simulink library "hal"  (Simulink 8.2)
settings: Solver=ode45  SolverMode=SingleTasking  StartTime=0.0  StopTime=10.0  RelTol=1e-3
PostLoadFcn:
  | , if any(exist('dsrtsu_mdlpostloadfcn', 'file') == [2, 3, 6]), try dsrtsu_mdlpostloadfcn('Execute', bdroot); catch fprintf('Error in PostLoadFcn (dsrtsu_mdlpostloadfcn) for model "%s":\n %s\n', bdroot, lasterr); end, end,
values from neighbouring files (symbols this model uses):
  INVALID_ABS1_TIMEOUT = single(0.03)    [hal_def.m]
  INVALID_ABS2_TIMEOUT = single(0.03)    [hal_def.m]
  INVALID_ABS3_TIMEOUT = single(0.03)    [hal_def.m]
  INVALID_ABS4_TIMEOUT = single(0.03)    [hal_def.m]
  INVALID_AC1_TIMEOUT = single(0.3)    [hal_def.m]
  INVALID_BCM1_TIMEOUT = single(0.6)    [hal_def.m]
  INVALID_BCM2_TIMEOUT = single(0.06)    [hal_def.m]
  INVALID_BOOSTER_VAC = uint32(255)    [hal_def.m]
  INVALID_CUR_VEHDECE = uint32(255)    [hal_def.m]
  INVALID_CURBRAKEDECE_REQ = uint32(255)    [hal_def.m]
  INVALID_CURSTEERANG_REQ = uint32(65535)    [hal_def.m]
  INVALID_CURSTEERTQ_REQ = uint32(255)    [hal_def.m]
  INVALID_ECM1_TIMEOUT = single(0.03)    [hal_def.m]
  INVALID_ECM2_TIMEOUT = single(0.03)    [hal_def.m]
  INVALID_ECM3_TIMEOUT = single(0.03)    [hal_def.m]
  INVALID_ECM9_TIMEOUT = single(0.03)    [hal_def.m]
  INVALID_ENG_TORQUE_FRICTIONAL = uint32(255)    [hal_def.m]
  INVALID_ENG_TORQUE_INDICATED = uint32(255)    [hal_def.m]
  INVALID_ENG_TORQUE_INDICATEDCOR = uint32(255)    [hal_def.m]
  INVALID_ENG_TQ_MAX = uint32(65535)    [hal_def.m]
  INVALID_ENG_TQ_MIN = uint32(65535)    [hal_def.m]
  INVALID_EPAS2_TIMEOUT = single(0.03)    [hal_def.m]
  INVALID_EPAS3_TIMEOUT = single(0.03)    [hal_def.m]
  INVALID_EPB1_TIMEOUT = single(0.12)    [hal_def.m]
  INVALID_EPS_BATTVOLT = uint32(251)    [hal_def.m]
  INVALID_ESC_BATTVOLT = uint32(251)    [hal_def.m]
  INVALID_GRADE = uint32(255)    [hal_def.m]
  INVALID_HCU3_TIMEOUT = single(0.03)    [hal_def.m]
  INVALID_HCU4_TIMEOUT = single(0.03)    [hal_def.m]
  INVALID_HMI1_TIMEOUT = single(0.03)    [hal_def.m]
  INVALID_HMI2_TIMEOUT = single(0.03)    [hal_def.m]
  INVALID_LAT_ACC = uint32(255)    [hal_def.m]
  INVALID_LONG_ACC = uint32(255)    [hal_def.m]
  INVALID_MC_PRESSURE = uint32(2047)    [hal_def.m]
  INVALID_METER1_TIMEOUT = single(0.3)    [hal_def.m]
  INVALID_METER3_TIMEOUT = single(0.3)    [hal_def.m]
  INVALID_METER_VEHSPD = uint32(2048)    [hal_def.m]
  INVALID_ODO_METER = uint32(1000000)    [hal_def.m]
  INVALID_OUTSIDE_TEMP = uint32(96)    [hal_def.m]
  INVALID_PARKBRAKEBIND_STAT = uint32(3)    [hal_def.m]
  INVALID_SAS1_TIMEOUT = single(0.03)    [hal_def.m]
  INVALID_SAS_ANGLE = uint32(65535)    [hal_def.m]
  INVALID_SHIFTER_POSN = uint32(6)    [hal_def.m]
  INVALID_TCM1_TIMEOUT = single(0.03)    [hal_def.m]
  INVALID_TCM2_TIMEOUT = single(0.03)    [hal_def.m]
  INVALID_VCU1_TIMEOUT = single(0.03)    [hal_def.m]
  INVALID_VCU2_TIMEOUT = single(0.03)    [hal_def.m]
  INVALID_VEH_CRASH = uint32(15)    [hal_def.m]
  INVALID_VEH_SPD = uint32(2048)    [hal_def.m]
  INVALID_WHEEL_SPD = uint32(16377)    [hal_def.m]
  INVALID_YAW_RATE = uint32(2001)    [hal_def.m]
undefined symbols (not defined in the file or in its folder): C_TASK_5MS_S, FALSE, INVALID_CURPTTORQ_REQ, KHAL_MssgIdObj1_num, KHAL_MssgIdObj2_num, KHAL_MssgIdObjStatus_num, TRUE
libraries: simulink x92
(part 7 of 8)

== system hal/dHAL_IN/HAL_IN_VCU/BO__883_HCU3__8_VCU ==
  CAN1_Rx : Inport
  Bus Selector : BusSelector  OutputSignals=HCU3.EngTqIndPermMax,HCU3.EngTqIndPermMax_P,HCU3.HCU3RollCnt
  EngTqIndPermMax : Outport
  EngTqIndPermMax_P : Outport  Port=2
  HCU3RollCnt : Outport  Port=3
  wires:
  Bus Selector/1 -> EngTqIndPermMax/1  "<EngTqIndPermMax>"
  Bus Selector/3 -> HCU3RollCnt/1  "<HCU3RollCnt>"
  Bus Selector/2 -> EngTqIndPermMax_P/1  "<EngTqIndPermMax_P>"
  [CAN1_Rx] -> Bus Selector/1
  CAN1_Rx/1 -> [CAN1_Rx]

== system hal/dHAL_IN/HAL_IN_VCU/BO__899_HCU4__8_VCU ==
  CAN1_Rx : Inport
  Bus Selector : BusSelector  OutputSignals=HCU4.MILReq
  MILReq : Outport
  wires:
  Bus Selector/1 -> MILReq/1  "<MILReq>"
  CAN1_Rx/1 -> [CAN1_Rx]
  [CAN1_Rx] -> Bus Selector/1

== system hal/dHAL_IN/dHAL_IN_ABS/BO_864_ABS2_8_ABS ==
  CAN1_Rx : Inport
  Bitwise Operator : simulink/Logic and Bit Operations/Bitwise Operator  logicop=AND  UseBitMask=on  BitMask=bin2dec('11110000')  BitMaskRealWorld=Stored Integer
  Bus Selector : BusSelector  OutputSignals=ABS2.ABS_Active,ABS2.ABS_Failed,ABS2.BrkSw_Sta,ABS2.BrkSw_V,ABS2.EBD_Failed,ABS2.ESC_Active,ABS2.ESC_Failed,ABS2.HSA_Active,ABS2.HSA_Failed,ABS2.TCS_Active,ABS2.TCS_Enabled,ABS2.TCS_Failed,ABS2.VehSpeed,ABS2.VehSpeed_Checksum,ABS2.VehSpeed_LifeCount
  Bus Selector1 : BusSelector  OutputSignals=ABS2.RAW_Byte_2,ABS2.RAW_Byte_1
  ChecksumCalculation : Subsystem  TreatAsAtomicUnit=on
  IcM : Subsystem  TreatAsAtomicUnit=on
  ABS_Active : Outport
  ABS_Failed : Outport  Port=2
  BrkSw_Sta : Outport  Port=3
  BrkSw_V : Outport  Port=4
  EBD_Failed : Outport  Port=5
  ESC_Active : Outport  Port=6
  ESC_Failed : Outport  Port=7
  HSA_Active : Outport  Port=8
  HSA_Failed : Outport  Port=9
  TCS_Active : Outport  Port=10
  TCS_Enabled : Outport  Port=11
  TCS_Failed : Outport  Port=12
  VehSpeed : Outport  Port=13
  VehSpeed_raw : Outport  Port=14
  VehSpeed_LifeCount : Outport  Port=15
  VehSpeed_Checksum : Outport  Port=16
  Message_Checksum : Outport  Port=17
  wires:
  IcM/1(HighLowByte) -> VehSpeed_raw/1
  Bitwise Operator/1 -> IcM/1(LowByte)
  Bus Selector1/2 -> IcM/2(HighByte)  "<RAW_Byte_1>"
  Bus Selector1/1 -> Bitwise Operator/1  "<RAW_Byte_2>"
  [CAN1_Rx] -> Bus Selector1/1
  ChecksumCalculation/1(Message_Checksum) -> Message_Checksum/1
  [CAN1_Rx] -> ChecksumCalculation/1(CAN1_Rx)
  Bus Selector/15 -> VehSpeed_LifeCount/1  "<VehSpeed_LifeCount>"
  Bus Selector/14 -> VehSpeed_Checksum/1  "<VehSpeed_Checksum>"
  Bus Selector/13 -> VehSpeed/1  "<VehSpeed>"
  Bus Selector/12 -> TCS_Failed/1  "<TCS_Failed>"
  Bus Selector/11 -> TCS_Enabled/1  "<TCS_Enabled>"
  Bus Selector/10 -> TCS_Active/1  "<TCS_Active>"
  Bus Selector/9 -> HSA_Failed/1  "<HSA_Failed>"
  Bus Selector/8 -> HSA_Active/1  "<HSA_Active>"
  Bus Selector/7 -> ESC_Failed/1  "<ESC_Failed>"
  Bus Selector/6 -> ESC_Active/1  "<ESC_Active>"
  Bus Selector/5 -> EBD_Failed/1  "<EBD_Failed>"
  Bus Selector/4 -> BrkSw_V/1  "<BrkSw_V>"
  Bus Selector/3 -> BrkSw_Sta/1  "<BrkSw_Sta>"
  Bus Selector/2 -> ABS_Failed/1  "<ABS_Failed>"
  Bus Selector/1 -> ABS_Active/1  "<ABS_Active>"
  CAN1_Rx/1 -> [CAN1_Rx]
  [CAN1_Rx] -> Bus Selector/1

== system hal/dHAL_IN/dHAL_IN_ABS/BO__848_ABS1__8_ABS ==
  CAN1_Rx : Inport
  Bus Selector : BusSelector  OutputSignals=ABS1.BoosterVac,ABS1.BoosterVac_Failed,ABS1.BoosterVac_Sta,ABS1.BoosterVac_V,ABS1.GRADE,ABS1.GRADE_V,ABS1.TCSRollCnt
  Bus Selector1 : BusSelector  OutputSignals=ABS1.RAW_Byte_8,ABS1.RAW_Byte_7
  BoosterVac : Outport
  BoosterVac_raw : Outport  Port=2
  BoosterVac_V : Outport  Port=3
  BoosterVac_Sta : Outport  Port=4
  BoosterVac_Failed : Outport  Port=5
  GRADE : Outport  Port=6
  GRADE_raw : Outport  Port=7
  GRADE_V : Outport  Port=8
  TCSRollCnt : Outport  Port=9
  wires:
  Bus Selector1/2 -> GRADE_raw/1  "<RAW_Byte_7>"
  Bus Selector1/1 -> BoosterVac_raw/1  "<RAW_Byte_8>"
  [CAN1_Rx] -> Bus Selector1/1
  Bus Selector/7 -> TCSRollCnt/1  "<TCSRollCnt>"
  Bus Selector/6 -> GRADE_V/1  "<GRADE_V>"
  Bus Selector/5 -> GRADE/1  "<GRADE>"
  Bus Selector/4 -> BoosterVac_V/1  "<BoosterVac_V>"
  Bus Selector/3 -> BoosterVac_Sta/1  "<BoosterVac_Sta>"
  Bus Selector/2 -> BoosterVac_Failed/1  "<BoosterVac_Failed>"
  Bus Selector/1 -> BoosterVac/1  "<BoosterVac>"
  CAN1_Rx/1 -> [CAN1_Rx]
  [CAN1_Rx] -> Bus Selector/1

== system hal/dHAL_IN/dHAL_IN_ABS/BO__880_ABS3__8_ABS ==
  CAN1_Rx : Inport
  Bitwise Operator{,1..3} (4 alike) : simulink/Logic and Bit Operations/Bitwise Operator  logicop=AND  UseBitMask=on  BitMask=bin2dec('11111110')  BitMaskRealWorld=Stored Integer
  Bus Selector : BusSelector  OutputSignals=ABS3.LF_RawWhlSpeed,ABS3.LF_RawWhlSpeed_V,ABS3.LR_RawWhlSpeed,ABS3.LR_RawWhlSpeed_V,ABS3.RF_RawWhlSpeed,ABS3.RF_RawWhlSpeed_V,ABS3.RR_RawWhlSpeed,ABS3.RR_RawWhlSpeed_V
  Bus Selector1 : BusSelector  OutputSignals=ABS3.RAW_Byte_2,ABS3.RAW_Byte_1,ABS3.RAW_Byte_4,ABS3.RAW_Byte_3,ABS3.RAW_Byte_6,ABS3.RAW_Byte_5,ABS3.RAW_Byte_8,ABS3.RAW_Byte_7
  IcM : Subsystem  TreatAsAtomicUnit=on
  IcM1 : Subsystem  TreatAsAtomicUnit=on
  IcM2 : Subsystem  TreatAsAtomicUnit=on
  IcM3 : Subsystem  TreatAsAtomicUnit=on
  LF_RawWhlSpeed : Outport
  LF_RawWhlSpeed_raw : Outport  Port=2
  LF_RawWhlSpeed_V : Outport  Port=3
  LR_RawWhlSpeed : Outport  Port=4
  LR_RawWhlSpeed_raw : Outport  Port=5
  LR_RawWhlSpeed_V : Outport  Port=6
  RF_RawWhlSpeed : Outport  Port=7
  RF_RawWhlSpeed_raw : Outport  Port=8
  RF_RawWhlSpeed_V : Outport  Port=9
  RR_RawWhlSpeed : Outport  Port=10
  RR_RawWhlSpeed_raw : Outport  Port=11
  RR_RawWhlSpeed_V : Outport  Port=12
  wires:
  IcM3/1(HighLowByte) -> LF_RawWhlSpeed_raw/1
  IcM2/1(HighLowByte) -> RF_RawWhlSpeed_raw/1
  Bus Selector1/8 -> IcM3/2(HighByte)  "<RAW_Byte_7>"
  Bus Selector1/7 -> Bitwise Operator3/1  "<RAW_Byte_8>"
  Bus Selector1/6 -> IcM2/2(HighByte)  "<RAW_Byte_5>"
  Bus Selector1/5 -> Bitwise Operator2/1  "<RAW_Byte_6>"
  Bitwise Operator3/1 -> IcM3/1(LowByte)
  Bitwise Operator2/1 -> IcM2/1(LowByte)
  Bus Selector1/4 -> IcM1/2(HighByte)  "<RAW_Byte_3>"
  Bus Selector1/3 -> Bitwise Operator1/1  "<RAW_Byte_4>"
  IcM1/1(HighLowByte) -> LR_RawWhlSpeed_raw/1
  Bitwise Operator1/1 -> IcM1/1(LowByte)
  Bus Selector1/2 -> IcM/2(HighByte)  "<RAW_Byte_1>"
  Bus Selector1/1 -> Bitwise Operator/1  "<RAW_Byte_2>"
  IcM/1(HighLowByte) -> RR_RawWhlSpeed_raw/1
  Bitwise Operator/1 -> IcM/1(LowByte)
  [CAN1_Rx] -> Bus Selector1/1
  Bus Selector/8 -> RR_RawWhlSpeed_V/1  "<RR_RawWhlSpeed_V>"
  Bus Selector/7 -> RR_RawWhlSpeed/1  "<RR_RawWhlSpeed>"
  Bus Selector/6 -> RF_RawWhlSpeed_V/1  "<RF_RawWhlSpeed_V>"
  Bus Selector/5 -> RF_RawWhlSpeed/1  "<RF_RawWhlSpeed>"
  Bus Selector/4 -> LR_RawWhlSpeed_V/1  "<LR_RawWhlSpeed_V>"
  Bus Selector/3 -> LR_RawWhlSpeed/1  "<LR_RawWhlSpeed>"
  Bus Selector/2 -> LF_RawWhlSpeed_V/1  "<LF_RawWhlSpeed_V>"
  Bus Selector/1 -> LF_RawWhlSpeed/1  "<LF_RawWhlSpeed>"
  [CAN1_Rx] -> Bus Selector/1
  CAN1_Rx/1 -> [CAN1_Rx]

== system hal/dHAL_IN/dHAL_IN_ABS/BO__896_ABS4__8_ABS ==
  CAN1_Rx : Inport
  Bitwise Operator : simulink/Logic and Bit Operations/Bitwise Operator  logicop=AND  UseBitMask=on  BitMask=bin2dec('00000111')  BitMaskRealWorld=Stored Integer
  Bus Selector : BusSelector  OutputSignals=ABS4.LatAccel,ABS4.LatAccel_V,ABS4.LongAccel,ABS4.LongAccel_V,ABS4.MCPressure,ABS4.MCPressure_V,ABS4.YawRate,ABS4.YawRate_V
  Bus Selector1 : BusSelector  OutputSignals=ABS4.RAW_Byte_3,ABS4.RAW_Byte_8,ABS4.RAW_Byte_5,ABS4.RAW_Byte_4
  Bus Selector2 : BusSelector  OutputSignals=ABS4.RAW_Byte_2,ABS4.RAW_Byte_1
  IcM : Subsystem  TreatAsAtomicUnit=on
  IcM1 : Subsystem  TreatAsAtomicUnit=on
  LatAccel : Outport
  LatAccel_raw : Outport  Port=2
  LatAccel_V : Outport  Port=3
  LongAccel : Outport  Port=4
  LongAcce_raw : Outport  Port=5
  LongAccel_V : Outport  Port=6
  MCPressure : Outport  Port=7
  MCPressure_raw : Outport  Port=8
  MCPressure_V : Outport  Port=9
  YawRate : Outport  Port=10
  YawRate_raw : Outport  Port=11
  YawRate_V : Outport  Port=12
  wires:
  Bitwise Operator/1 -> IcM1/2(HighByte)
  Bus Selector2/2 -> Bitwise Operator/1  "<RAW_Byte_1>"
  Bus Selector2/1 -> IcM1/1(LowByte)  "<RAW_Byte_2>"
  IcM/1(HighLowByte) -> YawRate_raw/1
  IcM1/1(HighLowByte) -> MCPressure_raw/1
  [CAN1_Rx] -> Bus Selector2/1
  Bus Selector1/4 -> IcM/2(HighByte)  "<RAW_Byte_4>"
  Bus Selector1/3 -> IcM/1(LowByte)  "<RAW_Byte_5>"
  Bus Selector1/2 -> LongAcce_raw/1  "<RAW_Byte_8>"
  Bus Selector1/1 -> LatAccel_raw/1  "<RAW_Byte_3>"
  [CAN1_Rx] -> Bus Selector1/1
  Bus Selector/8 -> YawRate_V/1  "<YawRate_V>"
  Bus Selector/7 -> YawRate/1  "<YawRate>"
  Bus Selector/6 -> MCPressure_V/1  "<MCPressure_V>"
  Bus Selector/5 -> MCPressure/1  "<MCPressure>"
  Bus Selector/4 -> LongAccel_V/1  "<LongAccel_V>"
  Bus Selector/3 -> LongAccel/1  "<LongAccel>"
  Bus Selector/2 -> LatAccel_V/1  "<LatAccel_V>"
  Bus Selector/1 -> LatAccel/1  "<LatAccel>"
  [CAN1_Rx] -> Bus Selector/1
  CAN1_Rx/1 -> [CAN1_Rx]

== system hal/dHAL_IN/dHAL_IN_AC/BO__1120_AC1__8_AC ==
  CAN1_Rx : Inport
  Bus Selector : BusSelector  OutputSignals=AC1.Sta_Out_Temp
  Bus Selector1 : BusSelector  OutputSignals=AC1.RAW_Byte_8
  Sta_Out_Temp : Outport
  Sta_Out_Temp_raw : Outport  Port=2
  wires:
  Bus Selector1/1 -> Sta_Out_Temp_raw/1  "<RAW_Byte_8>"
  Bus Selector/1 -> Sta_Out_Temp/1  "<Sta_Out_Temp>"
  [CAN1_Rx] -> Bus Selector1/1
  CAN1_Rx/1 -> [CAN1_Rx]
  [CAN1_Rx] -> Bus Selector/1

== system hal/dHAL_IN/dHAL_IN_BCM/BO__1008_BCM2__8_BCM ==
  CAN1_Rx : Inport
  Bus Selector : BusSelector  OutputSignals=BCM2.BCM_SRS_Crash_Info
  BCM_SRS_Crash_Info : Outport
  wires:
  Bus Selector/1 -> BCM_SRS_Crash_Info/1  "<BCM_SRS_Crash_Info>"
  CAN1_Rx/1 -> [CAN1_Rx]
  [CAN1_Rx] -> Bus Selector/1

== system hal/dHAL_IN/dHAL_IN_BCM/BO__1056_BCM1__8_BCM ==
  CAN1_Rx : Inport
  Bus Selector : BusSelector  OutputSignals=BCM1.BCM_AllDrSw_Sta,BCM1.BCM_DDrSw_Sta,BCM1.BCM_Hazard_Sta,BCM1.BCM_Key_Sta,BCM1.BCM_LRDrSw_Sta,BCM1.BCM_LTurnLp_Sta,BCM1.BCM_PDrSw_Sta,BCM1.BCM_RRDrSw_Sta,BCM1.BCM_RTurnLp_Sta,BCM1.BCM_TGateSw_Sta
  BCM_AllDrSw_Sta : Outport
  BCM_DDrSw_Sta : Outport  Port=2
  BCM_Hazard_Sta : Outport  Port=3
  BCM_Key_Sta : Outport  Port=4
  BCM_LRDrSw_Sta : Outport  Port=5
  BCM_LTurnLp_Sta : Outport  Port=6
  BCM_PDrSw_Sta : Outport  Port=7
  BCM_RRDrSw_Sta : Outport  Port=8
  BCM_RTurnLp_Sta : Outport  Port=9
  BCM_TGateSw_Sta : Outport  Port=10
  wires:
  Bus Selector/10 -> BCM_TGateSw_Sta/1  "<BCM_TGateSw_Sta>"
  Bus Selector/9 -> BCM_RTurnLp_Sta/1  "<BCM_RTurnLp_Sta>"
  Bus Selector/8 -> BCM_RRDrSw_Sta/1  "<BCM_RRDrSw_Sta>"
  Bus Selector/7 -> BCM_PDrSw_Sta/1  "<BCM_PDrSw_Sta>"
  Bus Selector/6 -> BCM_LTurnLp_Sta/1  "<BCM_LTurnLp_Sta>"
  Bus Selector/5 -> BCM_LRDrSw_Sta/1  "<BCM_LRDrSw_Sta>"
  Bus Selector/4 -> BCM_Key_Sta/1  "<BCM_Key_Sta>"
  Bus Selector/3 -> BCM_Hazard_Sta/1  "<BCM_Hazard_Sta>"
  Bus Selector/2 -> BCM_DDrSw_Sta/1  "<BCM_DDrSw_Sta>"
  Bus Selector/1 -> BCM_AllDrSw_Sta/1  "<BCM_AllDrSw_Sta>"
  [CAN1_Rx] -> Bus Selector/1
  CAN1_Rx/1 -> [CAN1_Rx]

== system hal/dHAL_IN/dHAL_IN_ECM/BO_790_ECM1_8_ECM ==
  CAN1_Rx : Inport
  Bus Selector : BusSelector  OutputSignals=ECM1.CAN_N,ECM1.CAN_TQFR,ECM1.CAN_TQI,ECM1.CAN_TQI_ACOR,ECM1.CAN_TQ_STND,ECM1.LV_CAN_N_ERR,ECM1.LV_CAN_SUB_TQI
  Bus Selector1 : BusSelector  OutputSignals=ECM1.RAW_Byte_6,ECM1.RAW_Byte_5,ECM1.RAW_Byte_2
  CAN_N : Outport
  CAN_TQFR : Outport  Port=2
  CAN_TQFR_raw : Outport  Port=3
  CAN_TQI : Outport  Port=4
  CAN_TQI_raw : Outport  Port=5
  CAN_TQI_ACOR : Outport  Port=6
  CAN_TQI_ACOR_raw : Outport  Port=7
  CAN_TQ_STND : Outport  Port=8
  LV_CAN_N_ERR : Outport  Port=9
  LV_CAN_SUB_TQI : Outport  Port=10
  wires:
  [CAN1_Rx] -> Bus Selector1/1
  [CAN1_Rx] -> Bus Selector/1
  CAN1_Rx/1 -> [CAN1_Rx]
  Bus Selector1/3 -> CAN_TQI_ACOR_raw/1  "<RAW_Byte_2>"
  Bus Selector1/2 -> CAN_TQI_raw/1  "<RAW_Byte_5>"
  Bus Selector1/1 -> CAN_TQFR_raw/1  "<RAW_Byte_6>"
  Bus Selector/7 -> LV_CAN_SUB_TQI/1  "<LV_CAN_SUB_TQI>"
  Bus Selector/6 -> LV_CAN_N_ERR/1  "<LV_CAN_N_ERR>"
  Bus Selector/5 -> CAN_TQ_STND/1  "<CAN_TQ_STND>"
  Bus Selector/4 -> CAN_TQI_ACOR/1  "<CAN_TQI_ACOR>"
  Bus Selector/3 -> CAN_TQI/1  "<CAN_TQI>"
  Bus Selector/2 -> CAN_TQFR/1  "<CAN_TQFR>"
  Bus Selector/1 -> CAN_N/1  "<CAN_N>"

== system hal/dHAL_IN/dHAL_IN_ECM/BO_809_ECM2_8_ECM ==
  CAN1_Rx : Inport
  Bus Selector : BusSelector  OutputSignals=ECM2.Eng_Hood_SW,ECM2.LV_CAN_ENG_RUN_ST
  Eng_Hood_SW : Outport
  LV_CAN_ENG_RUN_ST : Outport  Port=2
  wires:
  Bus Selector/1 -> Eng_Hood_SW/1  "<Eng_Hood_SW>"
  Bus Selector/2 -> LV_CAN_ENG_RUN_ST/1  "<LV_CAN_ENG_RUN_ST>"
  CAN1_Rx/1 -> Bus Selector/1

== system hal/dHAL_IN/dHAL_IN_ECM/BO_821_ECM3_8_ECM ==
  CAN1_Rx : Inport
  Bus Selector : BusSelector  OutputSignals=ECM3.CAN_PV_AV,ECM3.CAN_PV_EFC,ECM3.LV_CAN_ERRPAS,ECM3.LV_CAN_ERRPVS,ECM3.LV_CAN_MAIN_CRU,ECM3.LV_CAN_MAIN_CRU_ER,ECM3.LV_CAN_SET_CRU,ECM3.LV_CAN_SET_CRU_ERR
  CAN_PV_AV : Outport
  CAN_PV_EFC : Outport  Port=2
  LV_CAN_ERRPAS : Outport  Port=3
  LV_CAN_ERRPVS : Outport  Port=4
  LV_CAN_MAIN_CRU : Outport  Port=5
  LV_CAN_MAIN_CRU_ER : Outport  Port=6
  LV_CAN_SET_CRU : Outport  Port=7
  LV_CAN_SET_CRU_ERR : Outport  Port=8
  wires:
  Bus Selector/8 -> LV_CAN_SET_CRU_ERR/1  "<LV_CAN_SET_CRU_ERR>"
  Bus Selector/7 -> LV_CAN_SET_CRU/1  "<LV_CAN_SET_CRU>"
  Bus Selector/6 -> LV_CAN_MAIN_CRU_ER/1  "<LV_CAN_MAIN_CRU_ER>"
  Bus Selector/5 -> LV_CAN_MAIN_CRU/1  "<LV_CAN_MAIN_CRU>"
  Bus Selector/4 -> LV_CAN_ERRPVS/1  "<LV_CAN_ERRPVS>"
  Bus Selector/3 -> LV_CAN_ERRPAS/1  "<LV_CAN_ERRPAS>"
  Bus Selector/2 -> CAN_PV_EFC/1  "<CAN_PV_EFC>"
  Bus Selector/1 -> CAN_PV_AV/1  "<CAN_PV_AV>"
  CAN1_Rx/1 -> Bus Selector/1

== system hal/dHAL_IN/dHAL_IN_ECM/BO_875_ECM9_8_ECM ==
  CAN1_Rx1 : Inport
  Bus Selector : BusSelector  OutputSignals=ECM9.ECM9RollCnt,ECM9.EMSHybridOpState,ECM9.EMSOpState,ECM9.EngTqMax,ECM9.EngTqMin
  Bus Selector1 : BusSelector  OutputSignals=ECM9.RAW_Byte_5,ECM9.RAW_Byte_4,ECM9.RAW_Byte_7,ECM9.RAW_Byte_6
  IcM : Subsystem  TreatAsAtomicUnit=on
  IcM1 : Subsystem  TreatAsAtomicUnit=on
  ECM9RollCnt : Outport
  EMSHybridOpState : Outport  Port=2
  EMSOpState : Outport  Port=3
  EngTqMax : Outport  Port=4
  EngTqMax_raw : Outport  Port=5
  EngTqMin : Outport  Port=6
  EngTqMin_raw : Outport  Port=7
  wires:
  [CAN1_Rx] -> Bus Selector1/1
  [CAN1_Rx] -> Bus Selector/1
  CAN1_Rx1/1 -> [CAN1_Rx]
  IcM1/1(HighLowByte) -> EngTqMin_raw/1
  IcM/1(HighLowByte) -> EngTqMax_raw/1
  Bus Selector1/4 -> IcM1/2(HighByte)  "<RAW_Byte_6>"
  Bus Selector1/3 -> IcM1/1(LowByte)  "<RAW_Byte_7>"
  Bus Selector1/2 -> IcM/2(HighByte)  "<RAW_Byte_4>"
  Bus Selector1/1 -> IcM/1(LowByte)  "<RAW_Byte_5>"
  Bus Selector/5 -> EngTqMin/1  "<EngTqMin>"
  Bus Selector/4 -> EngTqMax/1  "<EngTqMax>"
  Bus Selector/3 -> EMSOpState/1  "<EMSOpState>"
  Bus Selector/2 -> EMSHybridOpState/1  "<EMSHybridOpState>"
  Bus Selector/1 -> ECM9RollCnt/1  "<ECM9RollCnt>"

== system hal/dHAL_IN/dHAL_IN_EPAS/BO__1365_EPAS3__8_EPAS ==
  CAN1_Rx : Inport
  Bus Selector : BusSelector  OutputSignals=EPAS3.CurStrAngReq,EPAS3.CurStrTqReq_A,EPAS3.CurStrTqReq,EPAS3.CurStrTqReq_A,EPAS3.DriverStrIntd,EPAS3.DriverStrIntdLvl,EPAS3.EPSBattVolt,EPAS3.EPAS3_Checksum,EPAS3.EPAS3_LifeCount
  Bus Selector1 : BusSelector  OutputSignals=EPAS3.RAW_Byte_2,EPAS3.RAW_Byte_1,EPAS3.RAW_Byte_5,EPAS3.RAW_Byte_6
  ChecksumCalculation : Subsystem  TreatAsAtomicUnit=on
  IcM : Subsystem  TreatAsAtomicUnit=on
  CurStrAngReq : Outport
  CurStrAngReq_raw : Outport  Port=2
  CurStrAngReq_A : Outport  Port=3
  CurStrTqReq : Outport  Port=4
  CurStrTqReq_raw : Outport  Port=5
  CurStrTqReq_A : Outport  Port=6
  DriverStrIntd : Outport  Port=7
  DriverStrIntdLvl : Outport  Port=8
  EPAS3_LifeCount : Outport  Port=9
  EPSBattVolt : Outport  Port=10
  EPSBattVolt_raw : Outport  Port=11
  EPAS3_Checksum : Outport  Port=12
  Message_Checksum : Outport  Port=13
  wires:
  Bus Selector1/4 -> EPSBattVolt_raw/1  "<RAW_Byte_6>"
  Bus Selector1/3 -> CurStrTqReq_raw/1  "<RAW_Byte_5>"
  IcM/1(HighLowByte) -> CurStrAngReq_raw/1
  Bus Selector1/2 -> IcM/2(HighByte)  "<RAW_Byte_1>"
  Bus Selector1/1 -> IcM/1(LowByte)  "<RAW_Byte_2>"
  Bus Selector/4 -> CurStrTqReq_A/1  "<CurStrTqReq_A>"
  Bus Selector/2 -> CurStrAngReq_A/1  "<CurStrTqReq_A>"
  ChecksumCalculation/1(Message_Checksum) -> Message_Checksum/1
  Bus Selector/7 -> EPSBattVolt/1  "<EPSBattVolt>"
  Bus Selector/9 -> ChecksumCalculation/1(EPAS3_LifeCount), EPAS3_LifeCount/1  "<EPAS3_LifeCount>"
  Bus Selector/8 -> EPAS3_Checksum/1  "<EPAS3_Checksum>"
  Bus Selector/6 -> DriverStrIntdLvl/1  "<DriverStrIntdLvl>"
  Bus Selector/5 -> DriverStrIntd/1  "<DriverStrIntd>"
  Bus Selector/3 -> CurStrTqReq/1  "<CurStrTqReq>"
  Bus Selector/1 -> CurStrAngReq/1  "<CurStrAngReq>"
  [CAN1_Rx] -> Bus Selector/1
  CAN1_Rx/1 -> [CAN1_Rx]
  [CAN1_Rx] -> ChecksumCalculation/2(CAN1_Rx)
  [CAN1_Rx] -> Bus Selector1/1

== system hal/dHAL_IN/dHAL_IN_EPAS/BO__922_SAS1__8_EPAS ==
  CAN1_Rx : Inport
  Bus Selector : BusSelector  OutputSignals=SAS1.SAS_Angle,SAS1.SAS_CAL,SAS1.SAS_CheckSum,SAS1.SAS_OK,SAS1.SAS_MsgCount
  Bus Selector1 : BusSelector  OutputSignals=SAS1.RAW_Byte_2,SAS1.RAW_Byte_1
  ChecksumCalculation : Subsystem  TreatAsAtomicUnit=on
  IcM : Subsystem  TreatAsAtomicUnit=on
  SAS_Angle : Outport
  SAS_Angle_raw : Outport  Port=2
  SAS_CAL : Outport  Port=3
  SAS_OK : Outport  Port=4
  SAS_MsgCount : Outport  Port=5
  SAS_CheckSum : Outport  Port=6
  Message_Checksum : Outport  Port=7
  wires:
  IcM/1(HighLowByte) -> SAS_Angle_raw/1
  Bus Selector1/2 -> IcM/2(HighByte)  "<RAW_Byte_1>"
  Bus Selector1/1 -> IcM/1(LowByte)  "<RAW_Byte_2>"
  [CAN1_Rx] -> Bus Selector1/1
  [CAN1_Rx] -> ChecksumCalculation/2(CAN1_Rx)
  ChecksumCalculation/1(Message_Checksum) -> Message_Checksum/1
  Bus Selector/4 -> SAS_OK/1  "<SAS_OK>"
  Bus Selector/5 -> ChecksumCalculation/1(SAS_MsgCount), SAS_MsgCount/1  "<SAS_MsgCount>"
  Bus Selector/3 -> SAS_CheckSum/1  "<SAS_CheckSum>"
  Bus Selector/2 -> SAS_CAL/1  "<SAS_CAL>"
  Bus Selector/1 -> SAS_Angle/1  "<SAS_Angle>"
  [CAN1_Rx] -> Bus Selector/1
  CAN1_Rx/1 -> [CAN1_Rx]

== system hal/dHAL_IN/dHAL_IN_EPAS/BO__926_EPAS2__8_EPAS ==
  CAN1_Rx : Inport
  Bus Selector : BusSelector  OutputSignals=EPAS2.Elect_PWR_Consumpt,EPAS2.EpasFailed,EPAS2.RSP_OK,EPAS2.R_SAS_Angle,EPAS2.Steering_Torque,EPAS2.Steering_Torque_V,EPAS2.SAS_CheckSum2,EPAS2.SAS_MsgCount2
  Bus Selector1 : BusSelector  OutputSignals=EPAS2.RAW_Byte_5,EPAS2.RAW_Byte_4
  ChecksumCalculation : Subsystem  TreatAsAtomicUnit=on
  IcM : Subsystem  TreatAsAtomicUnit=on
  Elect_PWR_Consumpt : Outport
  EpasFailed : Outport  Port=2
  R_SAS_Angle : Outport  Port=3
  R_SAS_Angle_raw : Outport  Port=4
  RSP_OK : Outport  Port=5
  SAS_MsgCount2 : Outport  Port=6
  Steering_Torque : Outport  Port=7
  Steering_Torque_V : Outport  Port=8
  SAS_CheckSum2 : Outport  Port=9
  Message_Checksum : Outport  Port=10
  wires:
  IcM/1(HighLowByte) -> R_SAS_Angle_raw/1
  Bus Selector1/2 -> IcM/2(HighByte)  "<RAW_Byte_4>"
  Bus Selector1/1 -> IcM/1(LowByte)  "<RAW_Byte_5>"
  [CAN1_Rx] -> Bus Selector1/1
  [CAN1_Rx] -> ChecksumCalculation/2(CAN1_Rx)
  ChecksumCalculation/1(Message_Checksum) -> Message_Checksum/1
  Bus Selector/6 -> Steering_Torque_V/1  "<Steering_Torque_V>"
  Bus Selector/5 -> Steering_Torque/1  "<Steering_Torque>"
  Bus Selector/8 -> SAS_MsgCount2/1, ChecksumCalculation/1(SAS_MsgCount)  "<SAS_MsgCount2>"
  Bus Selector/7 -> SAS_CheckSum2/1  "<SAS_CheckSum2>"
  Bus Selector/4 -> R_SAS_Angle/1  "<R_SAS_Angle>"
  Bus Selector/3 -> RSP_OK/1  "<RSP_OK>"
  Bus Selector/2 -> EpasFailed/1  "<EpasFailed>"
  Bus Selector/1 -> Elect_PWR_Consumpt/1  "<Elect_PWR_Consumpt>"
  CAN1_Rx/1 -> [CAN1_Rx]
  [CAN1_Rx] -> Bus Selector/1

== system hal/dHAL_IN/dHAL_IN_METER/BO__1104_Meter1__8_Meter ==
  CAN1_Rx : Inport
  Bus Selector : BusSelector  OutputSignals=Meter1.LowBrakeFluid_Sta,Meter1.ODOMETER,Meter1.ParkBrake,Meter1.SeatBelt
  LowBrakeFluid_Sta : Outport
  ODOMETER : Outport  Port=2
  ParkBrake : Outport  Port=3
  SeatBelt : Outport  Port=4
  wires:
  Bus Selector/1 -> LowBrakeFluid_Sta/1  "<LowBrakeFluid_Sta>"
  Bus Selector/2 -> ODOMETER/1  "<ODOMETER>"
  Bus Selector/3 -> ParkBrake/1  "<ParkBrake>"
  Bus Selector/4 -> SeatBelt/1  "<SeatBelt>"
  [CAN1_Rx] -> Bus Selector/1
  CAN1_Rx/1 -> [CAN1_Rx]

== system hal/dHAL_IN/dHAL_IN_METER/BO__1306_Meter3__8_Meter ==
  CAN1_Rx : Inport
  Bitwise Operator : simulink/Logic and Bit Operations/Bitwise Operator  logicop=AND  UseBitMask=on  BitMask=bin2dec('11110000')  BitMaskRealWorld=Stored Integer
  Bus Selector : BusSelector  OutputSignals=Meter3.Meter_Ind_VehSpeed
  Bus Selector1 : BusSelector  OutputSignals=Meter3.RAW_Byte_2,Meter3.RAW_Byte_1
  IcM : Subsystem  TreatAsAtomicUnit=on
  Meter_Ind_VehSpeed : Outport
  Meter_Ind_VehSpeed_raw : Outport  Port=2
  wires:
  Bus Selector1/2 -> IcM/2(HighByte)  "<RAW_Byte_1>"
  Bus Selector1/1 -> Bitwise Operator/1  "<RAW_Byte_2>"
  IcM/1(HighLowByte) -> Meter_Ind_VehSpeed_raw/1
  Bitwise Operator/1 -> IcM/1(LowByte)
  [CAN1_Rx] -> Bus Selector1/1
  Bus Selector/1 -> Meter_Ind_VehSpeed/1  "<Meter_Ind_VehSpeed>"
  CAN1_Rx/1 -> [CAN1_Rx]
  [CAN1_Rx] -> Bus Selector/1

== system hal/dHAL_IN/dHAL_IN_TCM/BO__832_TCM1__8_TCM ==
  CAN1_Rx : Inport
  Bus Selector : BusSelector  OutputSignals=TCM1.CAN_ETCU_STATE,TCM1.CAN_GEAR_SEL_ETCU,TCM1.CAN_GEAR_STATE_NOW,TCM1.CAN_GEAR_STA_NOW_V,TCM1.CAN_N_TM,TCM1.LV_CAN_N_TM_ERR
  CAN_ETCU_STATE : Outport
  CAN_GEAR_SEL_ETCU : Outport  Port=2
  CAN_GEAR_STATE_NOW : Outport  Port=3
  CAN_GEAR_STA_NOW_V : Outport  Port=4
  CAN_N_TM : Outport  Port=5
  LV_CAN_N_TM_ERR : Outport  Port=6
  wires:
  Bus Selector/6 -> LV_CAN_N_TM_ERR/1  "<LV_CAN_N_TM_ERR>"
  Bus Selector/5 -> CAN_N_TM/1  "<CAN_N_TM>"
  Bus Selector/4 -> CAN_GEAR_STA_NOW_V/1  "<CAN_GEAR_STA_NOW_V>"
  Bus Selector/3 -> CAN_GEAR_STATE_NOW/1  "<CAN_GEAR_STATE_NOW>"
  Bus Selector/2 -> CAN_GEAR_SEL_ETCU/1  "<CAN_GEAR_SEL_ETCU>"
  Bus Selector/1 -> CAN_ETCU_STATE/1  "<CAN_ETCU_STATE>"
  [CAN1_Rx] -> Bus Selector/1
  CAN1_Rx/1 -> [CAN1_Rx]

== system hal/dHAL_IN/dHAL_IN_TCM/BO__842_TCM2__8_TCM ==
  CAN1_Rx : Inport
  Bus Selector : BusSelector  OutputSignals=TCM2.DR_MODE_IND
  DR_MODE_IND : Outport
  wires:
  Bus Selector/1 -> DR_MODE_IND/1  "<DR_MODE_IND>"
  CAN1_Rx/1 -> [CAN1_Rx]
  [CAN1_Rx] -> Bus Selector/1

== system hal/dHAL_IN/HAL_IN_CANVALID/ChaekCANValid/Timer ==
  Enable : EnablePort  StatesWhenEnabling=reset  ZeroCross=off
  Constant : Constant  Value=C_TASK_5MS_S
  Sum : Sum  Inputs=|++  SaturateOnIntegerOverflow=on  InputSameDT=on
  Unit Delay : UnitDelay  SampleTime=-1
  Timer (sec) : Outport  OutputWhenDisabled=reset  InitialOutput=0
  wires:
  Constant/1 -> Sum/1
  Sum/1 -> Unit Delay/1
  Unit Delay/1 -> Sum/2, Timer (sec)/1

== system hal/dHAL_IN/HAL_IN_CANVALID/ChaekCANValid1/Timer ==
  Enable : EnablePort  StatesWhenEnabling=reset  ZeroCross=off
  Constant : Constant  Value=C_TASK_5MS_S
  Sum : Sum  Inputs=|++  SaturateOnIntegerOverflow=on  InputSameDT=on
  Unit Delay : UnitDelay  SampleTime=-1
  Timer (sec) : Outport  OutputWhenDisabled=reset  InitialOutput=0
  wires:
  Unit Delay/1 -> Timer (sec)/1, Sum/2
  Sum/1 -> Unit Delay/1
  Constant/1 -> Sum/1

== system hal/dHAL_IN/HAL_IN_CANVALID/ChaekCANValid10/Timer ==
  Enable : EnablePort  StatesWhenEnabling=reset  ZeroCross=off
  Constant : Constant  Value=C_TASK_5MS_S
  Sum : Sum  Inputs=|++  SaturateOnIntegerOverflow=on  InputSameDT=on
  Unit Delay : UnitDelay  SampleTime=-1
  Timer (sec) : Outport  OutputWhenDisabled=reset  InitialOutput=0
  wires:
  Unit Delay/1 -> Timer (sec)/1, Sum/2
  Sum/1 -> Unit Delay/1
  Constant/1 -> Sum/1

== system hal/dHAL_IN/HAL_IN_CANVALID/ChaekCANValid11/Timer ==
  Enable : EnablePort  StatesWhenEnabling=reset  ZeroCross=off
  Constant : Constant  Value=C_TASK_5MS_S
  Sum : Sum  Inputs=|++  SaturateOnIntegerOverflow=on  InputSameDT=on
  Unit Delay : UnitDelay  SampleTime=-1
  Timer (sec) : Outport  OutputWhenDisabled=reset  InitialOutput=0
  wires:
  Constant/1 -> Sum/1
  Sum/1 -> Unit Delay/1
  Unit Delay/1 -> Sum/2, Timer (sec)/1

== system hal/dHAL_IN/HAL_IN_CANVALID/ChaekCANValid12/Timer ==
  Enable : EnablePort  StatesWhenEnabling=reset  ZeroCross=off
  Constant : Constant  Value=C_TASK_5MS_S
  Sum : Sum  Inputs=|++  SaturateOnIntegerOverflow=on  InputSameDT=on
  Unit Delay : UnitDelay  SampleTime=-1
  Timer (sec) : Outport  OutputWhenDisabled=reset  InitialOutput=0
  wires:
  Unit Delay/1 -> Timer (sec)/1, Sum/2
  Sum/1 -> Unit Delay/1
  Constant/1 -> Sum/1

== system hal/dHAL_IN/HAL_IN_CANVALID/ChaekCANValid13/Timer ==
  Enable : EnablePort  StatesWhenEnabling=reset  ZeroCross=off
  Constant : Constant  Value=C_TASK_5MS_S
  Sum : Sum  Inputs=|++  SaturateOnIntegerOverflow=on  InputSameDT=on
  Unit Delay : UnitDelay  SampleTime=-1
  Timer (sec) : Outport  OutputWhenDisabled=reset  InitialOutput=0
  wires:
  Constant/1 -> Sum/1
  Sum/1 -> Unit Delay/1
  Unit Delay/1 -> Sum/2, Timer (sec)/1

== system hal/dHAL_IN/HAL_IN_CANVALID/ChaekCANValid14/Timer ==
  Enable : EnablePort  StatesWhenEnabling=reset  ZeroCross=off
  Constant : Constant  Value=C_TASK_5MS_S
  Sum : Sum  Inputs=|++  SaturateOnIntegerOverflow=on  InputSameDT=on
  Unit Delay : UnitDelay  SampleTime=-1
  Timer (sec) : Outport  OutputWhenDisabled=reset  InitialOutput=0
  wires:
  Constant/1 -> Sum/1
  Sum/1 -> Unit Delay/1
  Unit Delay/1 -> Sum/2, Timer (sec)/1

== system hal/dHAL_IN/HAL_IN_CANVALID/ChaekCANValid15/Timer ==
  Enable : EnablePort  StatesWhenEnabling=reset  ZeroCross=off
  Constant : Constant  Value=C_TASK_5MS_S
  Sum : Sum  Inputs=|++  SaturateOnIntegerOverflow=on  InputSameDT=on
  Unit Delay : UnitDelay  SampleTime=-1
  Timer (sec) : Outport  OutputWhenDisabled=reset  InitialOutput=0
  wires:
  Unit Delay/1 -> Timer (sec)/1, Sum/2
  Sum/1 -> Unit Delay/1
  Constant/1 -> Sum/1

== system hal/dHAL_IN/HAL_IN_CANVALID/ChaekCANValid16/Timer ==
  Enable : EnablePort  StatesWhenEnabling=reset  ZeroCross=off
  Constant : Constant  Value=C_TASK_5MS_S
  Sum : Sum  Inputs=|++  SaturateOnIntegerOverflow=on  InputSameDT=on
  Unit Delay : UnitDelay  SampleTime=-1
  Timer (sec) : Outport  OutputWhenDisabled=reset  InitialOutput=0
  wires:
  Constant/1 -> Sum/1
  Sum/1 -> Unit Delay/1
  Unit Delay/1 -> Sum/2, Timer (sec)/1

== system hal/dHAL_IN/HAL_IN_CANVALID/ChaekCANValid17/Timer ==
  Enable : EnablePort  StatesWhenEnabling=reset  ZeroCross=off
  Constant : Constant  Value=C_TASK_5MS_S
  Sum : Sum  Inputs=|++  SaturateOnIntegerOverflow=on  InputSameDT=on
  Unit Delay : UnitDelay  SampleTime=-1
  Timer (sec) : Outport  OutputWhenDisabled=reset  InitialOutput=0
  wires:
  Constant/1 -> Sum/1
  Sum/1 -> Unit Delay/1
  Unit Delay/1 -> Sum/2, Timer (sec)/1

== system hal/dHAL_IN/HAL_IN_CANVALID/ChaekCANValid18/Timer ==
  Enable : EnablePort  StatesWhenEnabling=reset  ZeroCross=off
  Constant : Constant  Value=C_TASK_5MS_S
  Sum : Sum  Inputs=|++  SaturateOnIntegerOverflow=on  InputSameDT=on
  Unit Delay : UnitDelay  SampleTime=-1
  Timer (sec) : Outport  OutputWhenDisabled=reset  InitialOutput=0
  wires:
  Unit Delay/1 -> Timer (sec)/1, Sum/2
  Sum/1 -> Unit Delay/1
  Constant/1 -> Sum/1

== system hal/dHAL_IN/HAL_IN_CANVALID/ChaekCANValid19/Timer ==
  Enable : EnablePort  StatesWhenEnabling=reset  ZeroCross=off
  Constant : Constant  Value=C_TASK_5MS_S
  Sum : Sum  Inputs=|++  SaturateOnIntegerOverflow=on  InputSameDT=on
  Unit Delay : UnitDelay  SampleTime=-1
  Timer (sec) : Outport  OutputWhenDisabled=reset  InitialOutput=0
  wires:
  Constant/1 -> Sum/1
  Sum/1 -> Unit Delay/1
  Unit Delay/1 -> Sum/2, Timer (sec)/1

== system hal/dHAL_IN/HAL_IN_CANVALID/ChaekCANValid2/Timer ==
  Enable : EnablePort  StatesWhenEnabling=reset  ZeroCross=off
  Constant : Constant  Value=C_TASK_5MS_S
  Sum : Sum  Inputs=|++  SaturateOnIntegerOverflow=on  InputSameDT=on
  Unit Delay : UnitDelay  SampleTime=-1
  Timer (sec) : Outport  OutputWhenDisabled=reset  InitialOutput=0
  wires:
  Constant/1 -> Sum/1
  Sum/1 -> Unit Delay/1
  Unit Delay/1 -> Sum/2, Timer (sec)/1

== system hal/dHAL_IN/HAL_IN_CANVALID/ChaekCANValid20/Timer ==
  Enable : EnablePort  StatesWhenEnabling=reset  ZeroCross=off
  Constant : Constant  Value=C_TASK_5MS_S
  Sum : Sum  Inputs=|++  SaturateOnIntegerOverflow=on  InputSameDT=on
  Unit Delay : UnitDelay  SampleTime=-1
  Timer (sec) : Outport  OutputWhenDisabled=reset  InitialOutput=0
  wires:
  Unit Delay/1 -> Timer (sec)/1, Sum/2
  Sum/1 -> Unit Delay/1
  Constant/1 -> Sum/1

== system hal/dHAL_IN/HAL_IN_CANVALID/ChaekCANValid21/Timer ==
  Enable : EnablePort  StatesWhenEnabling=reset  ZeroCross=off
  Constant : Constant  Value=C_TASK_5MS_S
  Sum : Sum  Inputs=|++  SaturateOnIntegerOverflow=on  InputSameDT=on
  Unit Delay : UnitDelay  SampleTime=-1
  Timer (sec) : Outport  OutputWhenDisabled=reset  InitialOutput=0
  wires:
  Unit Delay/1 -> Timer (sec)/1, Sum/2
  Sum/1 -> Unit Delay/1
  Constant/1 -> Sum/1

== system hal/dHAL_IN/HAL_IN_CANVALID/ChaekCANValid22/Timer ==
  Enable : EnablePort  StatesWhenEnabling=reset  ZeroCross=off
  Constant : Constant  Value=C_TASK_5MS_S
  Sum : Sum  Inputs=|++  SaturateOnIntegerOverflow=on  InputSameDT=on
  Unit Delay : UnitDelay  SampleTime=-1
  Timer (sec) : Outport  OutputWhenDisabled=reset  InitialOutput=0
  wires:
  Constant/1 -> Sum/1
  Sum/1 -> Unit Delay/1
  Unit Delay/1 -> Sum/2, Timer (sec)/1

== system hal/dHAL_IN/HAL_IN_CANVALID/ChaekCANValid23/Timer ==
  Enable : EnablePort  StatesWhenEnabling=reset  ZeroCross=off
  Constant : Constant  Value=C_TASK_5MS_S
  Sum : Sum  Inputs=|++  SaturateOnIntegerOverflow=on  InputSameDT=on
  Unit Delay : UnitDelay  SampleTime=-1
  Timer (sec) : Outport  OutputWhenDisabled=reset  InitialOutput=0
  wires:
  Unit Delay/1 -> Timer (sec)/1, Sum/2
  Sum/1 -> Unit Delay/1
  Constant/1 -> Sum/1

== system hal/dHAL_IN/HAL_IN_CANVALID/ChaekCANValid24/Timer ==
  Enable : EnablePort  StatesWhenEnabling=reset  ZeroCross=off
  Constant : Constant  Value=C_TASK_5MS_S
  Sum : Sum  Inputs=|++  SaturateOnIntegerOverflow=on  InputSameDT=on
  Unit Delay : UnitDelay  SampleTime=-1
  Timer (sec) : Outport  OutputWhenDisabled=reset  InitialOutput=0
  wires:
  Unit Delay/1 -> Timer (sec)/1, Sum/2
  Sum/1 -> Unit Delay/1
  Constant/1 -> Sum/1

== system hal/dHAL_IN/HAL_IN_CANVALID/ChaekCANValid3/Timer ==
  Enable : EnablePort  StatesWhenEnabling=reset  ZeroCross=off
  Constant : Constant  Value=C_TASK_5MS_S
  Sum : Sum  Inputs=|++  SaturateOnIntegerOverflow=on  InputSameDT=on
  Unit Delay : UnitDelay  SampleTime=-1
  Timer (sec) : Outport  OutputWhenDisabled=reset  InitialOutput=0
  wires:
  Unit Delay/1 -> Timer (sec)/1, Sum/2
  Sum/1 -> Unit Delay/1
  Constant/1 -> Sum/1

== system hal/dHAL_IN/HAL_IN_CANVALID/ChaekCANValid4/Timer ==
  Enable : EnablePort  StatesWhenEnabling=reset  ZeroCross=off
  Constant : Constant  Value=C_TASK_5MS_S
  Sum : Sum  Inputs=|++  SaturateOnIntegerOverflow=on  InputSameDT=on
  Unit Delay : UnitDelay  SampleTime=-1
  Timer (sec) : Outport  OutputWhenDisabled=reset  InitialOutput=0
  wires:
  Constant/1 -> Sum/1
  Sum/1 -> Unit Delay/1
  Unit Delay/1 -> Sum/2, Timer (sec)/1

== system hal/dHAL_IN/HAL_IN_CANVALID/ChaekCANValid5/Timer ==
  Enable : EnablePort  StatesWhenEnabling=reset  ZeroCross=off
  Constant : Constant  Value=C_TASK_5MS_S
  Sum : Sum  Inputs=|++  SaturateOnIntegerOverflow=on  InputSameDT=on
  Unit Delay : UnitDelay  SampleTime=-1
  Timer (sec) : Outport  OutputWhenDisabled=reset  InitialOutput=0
  wires:
  Unit Delay/1 -> Timer (sec)/1, Sum/2
  Sum/1 -> Unit Delay/1
  Constant/1 -> Sum/1

== system hal/dHAL_IN/HAL_IN_CANVALID/ChaekCANValid6/Timer ==
  Enable : EnablePort  StatesWhenEnabling=reset  ZeroCross=off
  Constant : Constant  Value=C_TASK_5MS_S
  Sum : Sum  Inputs=|++  SaturateOnIntegerOverflow=on  InputSameDT=on
  Unit Delay : UnitDelay  SampleTime=-1
  Timer (sec) : Outport  OutputWhenDisabled=reset  InitialOutput=0
  wires:
  Constant/1 -> Sum/1
  Sum/1 -> Unit Delay/1
  Unit Delay/1 -> Sum/2, Timer (sec)/1

== system hal/dHAL_IN/HAL_IN_CANVALID/ChaekCANValid7/Timer ==
  Enable : EnablePort  StatesWhenEnabling=reset  ZeroCross=off
  Constant : Constant  Value=C_TASK_5MS_S
  Sum : Sum  Inputs=|++  SaturateOnIntegerOverflow=on  InputSameDT=on
  Unit Delay : UnitDelay  SampleTime=-1
  Timer (sec) : Outport  OutputWhenDisabled=reset  InitialOutput=0
  wires:
  Unit Delay/1 -> Timer (sec)/1, Sum/2
  Sum/1 -> Unit Delay/1
  Constant/1 -> Sum/1

== system hal/dHAL_IN/HAL_IN_CANVALID/ChaekCANValid8/Timer ==
  Enable : EnablePort  StatesWhenEnabling=reset  ZeroCross=off
  Constant : Constant  Value=C_TASK_5MS_S
  Sum : Sum  Inputs=|++  SaturateOnIntegerOverflow=on  InputSameDT=on
  Unit Delay : UnitDelay  SampleTime=-1
  Timer (sec) : Outport  OutputWhenDisabled=reset  InitialOutput=0
  wires:
  Unit Delay/1 -> Timer (sec)/1, Sum/2
  Sum/1 -> Unit Delay/1
  Constant/1 -> Sum/1

== system hal/dHAL_IN/HAL_IN_CANVALID/ChaekCANValid9/Timer ==
  Enable : EnablePort  StatesWhenEnabling=reset  ZeroCross=off
  Constant : Constant  Value=C_TASK_5MS_S
  Sum : Sum  Inputs=|++  SaturateOnIntegerOverflow=on  InputSameDT=on
  Unit Delay : UnitDelay  SampleTime=-1
  Timer (sec) : Outport  OutputWhenDisabled=reset  InitialOutput=0
  wires:
  Constant/1 -> Sum/1
  Sum/1 -> Unit Delay/1
  Unit Delay/1 -> Sum/2, Timer (sec)/1

== system hal/dHAL_IN/HAL_IN_RadObjDecoder/RObjectPackFrame/RObjects_Decoder_v2 ==
  Status : Inport
  ID : Inport  Port=2
  Byte1 : Inport  Port=3
  Byte2 : Inport  Port=4
  Byte3 : Inport  Port=5
  Byte4 : Inport  Port=6
  Byte5 : Inport  Port=7
  Byte6 : Inport  Port=8
  Byte7 : Inport  Port=9
  Byte8 : Inport  Port=10
  R_Objects_in : Inport  Port=11
  CheckIDs : Subsystem
  ParseFrames : Subsystem
  R_Objects_out : Outport  OutDataTypeStr=Bus: R_Objects
  wires:
  Byte8/1 -> ParseFrames/9(Byte8)
  Byte7/1 -> ParseFrames/8(Byte7)
  Byte6/1 -> ParseFrames/7(Byte6)
  Byte5/1 -> ParseFrames/6(Byte5)
  Byte4/1 -> ParseFrames/5(Byte4)
  [ParseFrame] -> ParseFrames/Trigger
  CheckIDs/2(ParseFrame) -> [ParseFrame]
  ParseFrames/1(R_Objects_out) -> R_Objects_out/1
  CheckIDs/1(R_Objects_out) -> ParseFrames/1(R_Objects_in)
  Byte3/1 -> ParseFrames/4(Byte3)
  Byte2/1 -> ParseFrames/3(Byte2)
  Byte1/1 -> ParseFrames/2(Byte1)
  R_Objects_in/1 -> CheckIDs/3(R_Objects_in)
  ID/1 -> CheckIDs/2(ID)
  Status/1 -> CheckIDs/1(Status)

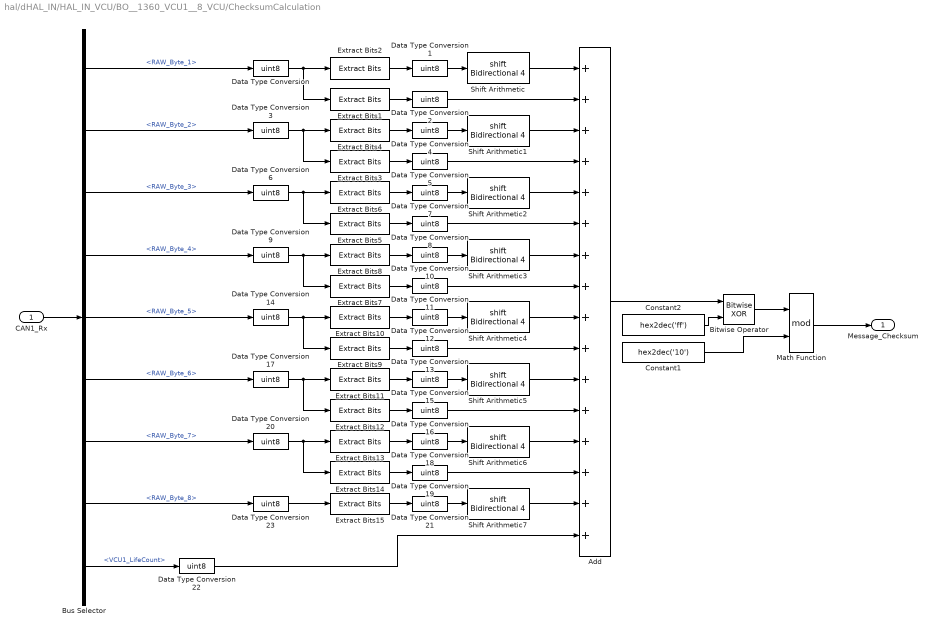
== system hal/dHAL_IN/HAL_IN_VCU/BO__1360_VCU1__8_VCU/ChecksumCalculation ==
  CAN1_Rx : Inport
  Add : Sum  Inputs=16
  Bitwise Operator : simulink/Logic and Bit Operations/Bitwise Operator  logicop=XOR  UseBitMask=off  NumInputPorts=2  BitMask=bin2dec('11011001')  BitMaskRealWorld=Stored Integer
  Bus Selector : BusSelector  OutputSignals=VCU1.RAW_Byte_1,VCU1.RAW_Byte_2,VCU1.RAW_Byte_3,VCU1.RAW_Byte_4,VCU1.RAW_Byte_5,VCU1.RAW_Byte_6,VCU1.RAW_Byte_7,VCU1.RAW_Byte_8,VCU1.VCU1_LifeCount
  Constant1 : Constant  Value=hex2dec('10')  OutDataTypeStr=uint8
  Constant2 : Constant  Value=hex2dec('ff')  OutDataTypeStr=uint8
  Data Type Conversion{,1..23} (24 alike) : DataTypeConversion  OutDataTypeStr=uint8
  Extract Bits{1,3,5,7,9,12,14} (7 alike) : simulink/Logic and Bit Operations/Extract Bits  bitsToExtract=Lower half  numBits=8  bitIdxRange=[0 7]  outScalingMode=Preserve fixed-point scaling
  Extract Bits{2,4,6,8,10..11,13,15} (8 alike) : simulink/Logic and Bit Operations/Extract Bits  bitsToExtract=Upper half  numBits=8  bitIdxRange=[0 7]  outScalingMode=Preserve fixed-point scaling
  Math Function : Math  Operator=mod  SaturateOnIntegerOverflow=on
  Shift Arithmetic{,1..7} (8 alike) : ArithShift  BitShiftNumber=4
  Message_Checksum : Outport
  wires:
  Bus Selector/9 -> Data Type Conversion22/1  "<VCU1_LifeCount>"
  CAN1_Rx/1 -> Bus Selector/1
  Math Function/1 -> Message_Checksum/1
  Constant1/1 -> Math Function/2
  Bitwise Operator/1 -> Math Function/1
  Constant2/1 -> Bitwise Operator/2
  Add/1 -> Bitwise Operator/1
  Data Type Conversion22/1 -> Add/16
  Bus Selector/8 -> Data Type Conversion23/1  "<RAW_Byte_8>"
  Shift Arithmetic7/1 -> Add/15
  Data Type Conversion23/1 -> Extract Bits15/1
  Data Type Conversion21/1 -> Shift Arithmetic7/1
  Extract Bits15/1 -> Data Type Conversion21/1
  Bus Selector/7 -> Data Type Conversion20/1  "<RAW_Byte_7>"
  Data Type Conversion19/1 -> Add/14
  Shift Arithmetic6/1 -> Add/13
  Data Type Conversion20/1 -> Extract Bits14/1, Extract Bits13/1
  Data Type Conversion18/1 -> Shift Arithmetic6/1
  Extract Bits14/1 -> Data Type Conversion19/1
  Extract Bits13/1 -> Data Type Conversion18/1
  Bus Selector/6 -> Data Type Conversion17/1  "<RAW_Byte_6>"
  Data Type Conversion16/1 -> Add/12
  Shift Arithmetic5/1 -> Add/11
  Data Type Conversion17/1 -> Extract Bits11/1, Extract Bits12/1
  Data Type Conversion15/1 -> Shift Arithmetic5/1
  Extract Bits12/1 -> Data Type Conversion16/1
  Extract Bits11/1 -> Data Type Conversion15/1
  Bus Selector/5 -> Data Type Conversion14/1  "<RAW_Byte_5>"
  Data Type Conversion13/1 -> Add/10
  Shift Arithmetic4/1 -> Add/9
  Data Type Conversion14/1 -> Extract Bits9/1, Extract Bits10/1
  Data Type Conversion12/1 -> Shift Arithmetic4/1
  Extract Bits9/1 -> Data Type Conversion13/1
  Extract Bits10/1 -> Data Type Conversion12/1
  Bus Selector/4 -> Data Type Conversion9/1  "<RAW_Byte_4>"
  Data Type Conversion11/1 -> Add/8
  Shift Arithmetic3/1 -> Add/7
  Data Type Conversion9/1 -> Extract Bits8/1, Extract Bits7/1
  Data Type Conversion10/1 -> Shift Arithmetic3/1
  Extract Bits7/1 -> Data Type Conversion11/1
  Extract Bits8/1 -> Data Type Conversion10/1
  Bus Selector/3 -> Data Type Conversion6/1  "<RAW_Byte_3>"
  Data Type Conversion8/1 -> Add/6
  Shift Arithmetic2/1 -> Add/5
  Data Type Conversion6/1 -> Extract Bits5/1, Extract Bits6/1
  Data Type Conversion7/1 -> Shift Arithmetic2/1
  Extract Bits5/1 -> Data Type Conversion8/1
  Extract Bits6/1 -> Data Type Conversion7/1
  Bus Selector/2 -> Data Type Conversion3/1  "<RAW_Byte_2>"
  Data Type Conversion5/1 -> Add/4
  Shift Arithmetic1/1 -> Add/3
  Data Type Conversion2/1 -> Add/2
  Shift Arithmetic/1 -> Add/1
  Data Type Conversion3/1 -> Extract Bits4/1, Extract Bits3/1
  Data Type Conversion4/1 -> Shift Arithmetic1/1
  Extract Bits3/1 -> Data Type Conversion5/1
  Extract Bits4/1 -> Data Type Conversion4/1
  Data Type Conversion/1 -> Extract Bits1/1, Extract Bits2/1
  Data Type Conversion1/1 -> Shift Arithmetic/1
  Extract Bits1/1 -> Data Type Conversion2/1
  Extract Bits2/1 -> Data Type Conversion1/1
  Bus Selector/1 -> Data Type Conversion/1  "<RAW_Byte_1>"

== system hal/dHAL_IN/HAL_IN_VCU/BO__1360_VCU1__8_VCU/IcM ==
  LowByte : Inport
  HighByte : Inport  Port=2
  Bitwise Operator : simulink/Logic and Bit Operations/Bitwise Operator  logicop=OR  UseBitMask=off  NumInputPorts=2  BitMask=bin2dec('11011001')  BitMaskRealWorld=Stored Integer
  Cast1 : DataTypeConversion  OutDataTypeStr=uint16  RndMeth=Zero
  Cast45 : DataTypeConversion  OutDataTypeStr=uint16  RndMeth=Zero
  Shift Arithmetic : ArithShift  BitShiftNumber=-4
  Shift Arithmetic1 : ArithShift  BitShiftNumber=4
  HighLowByte : Outport
  wires:
  Shift Arithmetic1/1 -> Bitwise Operator/2
  LowByte/1 -> Cast1/1
  Cast1/1 -> Shift Arithmetic1/1
  Cast45/1 -> Shift Arithmetic/1
  HighByte/1 -> Cast45/1
  Bitwise Operator/1 -> HighLowByte/1
  Shift Arithmetic/1 -> Bitwise Operator/1

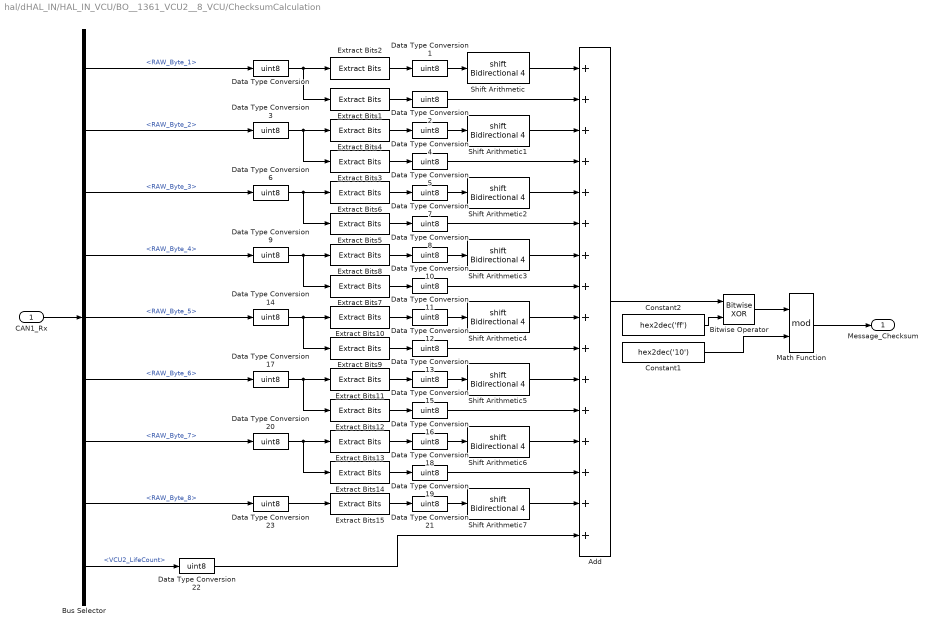
== system hal/dHAL_IN/HAL_IN_VCU/BO__1361_VCU2__8_VCU/ChecksumCalculation ==
  CAN1_Rx : Inport
  Add : Sum  Inputs=16
  Bitwise Operator : simulink/Logic and Bit Operations/Bitwise Operator  logicop=XOR  UseBitMask=off  NumInputPorts=2  BitMask=bin2dec('11011001')  BitMaskRealWorld=Stored Integer
  Bus Selector : BusSelector  OutputSignals=VCU2.RAW_Byte_1,VCU2.RAW_Byte_2,VCU2.RAW_Byte_3,VCU2.RAW_Byte_4,VCU2.RAW_Byte_5,VCU2.RAW_Byte_6,VCU2.RAW_Byte_7,VCU2.RAW_Byte_8,VCU2.VCU2_LifeCount
  Constant1 : Constant  Value=hex2dec('10')  OutDataTypeStr=uint8
  Constant2 : Constant  Value=hex2dec('ff')  OutDataTypeStr=uint8
  Data Type Conversion{,1..23} (24 alike) : DataTypeConversion  OutDataTypeStr=uint8
  Extract Bits{1,3,5,7,9,12,14} (7 alike) : simulink/Logic and Bit Operations/Extract Bits  bitsToExtract=Lower half  numBits=8  bitIdxRange=[0 7]  outScalingMode=Preserve fixed-point scaling
  Extract Bits{2,4,6,8,10..11,13,15} (8 alike) : simulink/Logic and Bit Operations/Extract Bits  bitsToExtract=Upper half  numBits=8  bitIdxRange=[0 7]  outScalingMode=Preserve fixed-point scaling
  Math Function : Math  Operator=mod  SaturateOnIntegerOverflow=on
  Shift Arithmetic{,1..7} (8 alike) : ArithShift  BitShiftNumber=4
  Message_Checksum : Outport
  wires:
  Bus Selector/9 -> Data Type Conversion22/1  "<VCU2_LifeCount>"
  CAN1_Rx/1 -> Bus Selector/1
  Math Function/1 -> Message_Checksum/1
  Constant1/1 -> Math Function/2
  Bitwise Operator/1 -> Math Function/1
  Constant2/1 -> Bitwise Operator/2
  Add/1 -> Bitwise Operator/1
  Data Type Conversion22/1 -> Add/16
  Bus Selector/8 -> Data Type Conversion23/1  "<RAW_Byte_8>"
  Shift Arithmetic7/1 -> Add/15
  Data Type Conversion23/1 -> Extract Bits15/1
  Data Type Conversion21/1 -> Shift Arithmetic7/1
  Extract Bits15/1 -> Data Type Conversion21/1
  Bus Selector/7 -> Data Type Conversion20/1  "<RAW_Byte_7>"
  Data Type Conversion19/1 -> Add/14
  Shift Arithmetic6/1 -> Add/13
  Data Type Conversion20/1 -> Extract Bits14/1, Extract Bits13/1
  Data Type Conversion18/1 -> Shift Arithmetic6/1
  Extract Bits14/1 -> Data Type Conversion19/1
  Extract Bits13/1 -> Data Type Conversion18/1
  Bus Selector/6 -> Data Type Conversion17/1  "<RAW_Byte_6>"
  Data Type Conversion16/1 -> Add/12
  Shift Arithmetic5/1 -> Add/11
  Data Type Conversion17/1 -> Extract Bits11/1, Extract Bits12/1
  Data Type Conversion15/1 -> Shift Arithmetic5/1
  Extract Bits12/1 -> Data Type Conversion16/1
  Extract Bits11/1 -> Data Type Conversion15/1
  Bus Selector/5 -> Data Type Conversion14/1  "<RAW_Byte_5>"
  Data Type Conversion13/1 -> Add/10
  Shift Arithmetic4/1 -> Add/9
  Data Type Conversion14/1 -> Extract Bits9/1, Extract Bits10/1
  Data Type Conversion12/1 -> Shift Arithmetic4/1
  Extract Bits9/1 -> Data Type Conversion13/1
  Extract Bits10/1 -> Data Type Conversion12/1
  Bus Selector/4 -> Data Type Conversion9/1  "<RAW_Byte_4>"
  Data Type Conversion11/1 -> Add/8
  Shift Arithmetic3/1 -> Add/7
  Data Type Conversion9/1 -> Extract Bits8/1, Extract Bits7/1
  Data Type Conversion10/1 -> Shift Arithmetic3/1
  Extract Bits7/1 -> Data Type Conversion11/1
  Extract Bits8/1 -> Data Type Conversion10/1
  Bus Selector/3 -> Data Type Conversion6/1  "<RAW_Byte_3>"
  Data Type Conversion8/1 -> Add/6
  Shift Arithmetic2/1 -> Add/5
  Data Type Conversion6/1 -> Extract Bits5/1, Extract Bits6/1
  Data Type Conversion7/1 -> Shift Arithmetic2/1
  Extract Bits5/1 -> Data Type Conversion8/1
  Extract Bits6/1 -> Data Type Conversion7/1
  Bus Selector/2 -> Data Type Conversion3/1  "<RAW_Byte_2>"
  Data Type Conversion5/1 -> Add/4
  Shift Arithmetic1/1 -> Add/3
  Data Type Conversion2/1 -> Add/2
  Shift Arithmetic/1 -> Add/1
  Data Type Conversion3/1 -> Extract Bits4/1, Extract Bits3/1
  Data Type Conversion4/1 -> Shift Arithmetic1/1
  Extract Bits3/1 -> Data Type Conversion5/1
  Extract Bits4/1 -> Data Type Conversion4/1
  Data Type Conversion/1 -> Extract Bits1/1, Extract Bits2/1
  Data Type Conversion1/1 -> Shift Arithmetic/1
  Extract Bits1/1 -> Data Type Conversion2/1
  Extract Bits2/1 -> Data Type Conversion1/1
  Bus Selector/1 -> Data Type Conversion/1  "<RAW_Byte_1>"

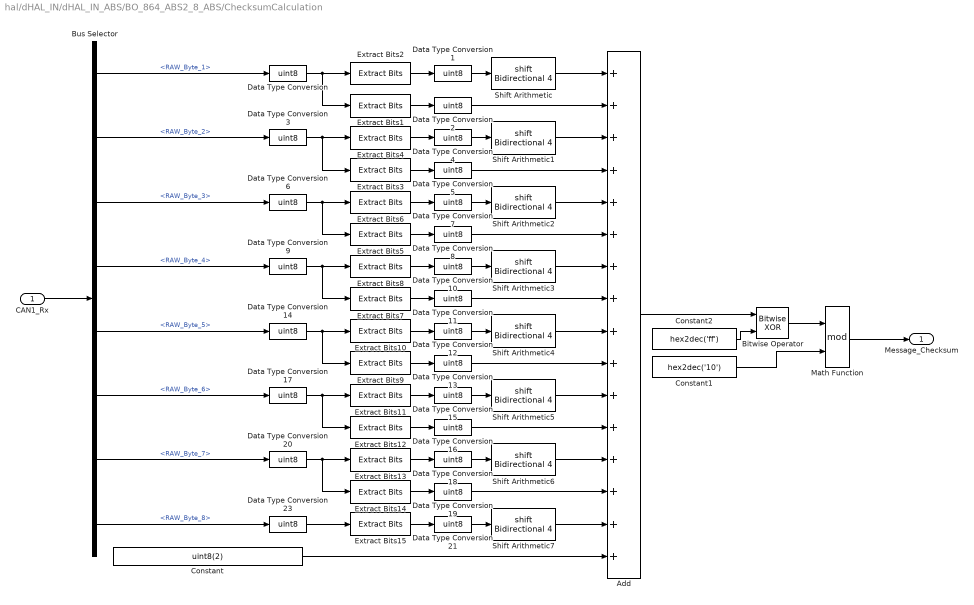
== system hal/dHAL_IN/dHAL_IN_ABS/BO_864_ABS2_8_ABS/ChecksumCalculation ==
  CAN1_Rx : Inport
  Add : Sum  Inputs=16
  Bitwise Operator : simulink/Logic and Bit Operations/Bitwise Operator  logicop=XOR  UseBitMask=off  NumInputPorts=2  BitMask=bin2dec('11011001')  BitMaskRealWorld=Stored Integer
  Bus Selector : BusSelector  OutputSignals=ABS2.RAW_Byte_1,ABS2.RAW_Byte_2,ABS2.RAW_Byte_3,ABS2.RAW_Byte_4,ABS2.RAW_Byte_5,ABS2.RAW_Byte_6,ABS2.RAW_Byte_7,ABS2.RAW_Byte_8
  Constant : Constant  Value=uint8(2)
  Constant1 : Constant  Value=hex2dec('10')  OutDataTypeStr=uint8
  Constant2 : Constant  Value=hex2dec('ff')  OutDataTypeStr=uint8
  Data Type Conversion{,1..21,23} (23 alike) : DataTypeConversion  OutDataTypeStr=uint8
  Extract Bits{1,3,5,7,9,12,14} (7 alike) : simulink/Logic and Bit Operations/Extract Bits  bitsToExtract=Lower half  numBits=8  bitIdxRange=[0 7]  outScalingMode=Preserve fixed-point scaling
  Extract Bits{2,4,6,8,10..11,13,15} (8 alike) : simulink/Logic and Bit Operations/Extract Bits  bitsToExtract=Upper half  numBits=8  bitIdxRange=[0 7]  outScalingMode=Preserve fixed-point scaling
  Math Function : Math  Operator=mod  SaturateOnIntegerOverflow=on
  Shift Arithmetic{,1..7} (8 alike) : ArithShift  BitShiftNumber=4
  Message_Checksum : Outport
  wires:
  CAN1_Rx/1 -> Bus Selector/1
  Math Function/1 -> Message_Checksum/1
  Constant1/1 -> Math Function/2
  Bitwise Operator/1 -> Math Function/1
  Constant2/1 -> Bitwise Operator/2
  Add/1 -> Bitwise Operator/1
  Constant/1 -> Add/16
  Bus Selector/8 -> Data Type Conversion23/1  "<RAW_Byte_8>"
  Shift Arithmetic7/1 -> Add/15
  Data Type Conversion23/1 -> Extract Bits15/1
  Data Type Conversion21/1 -> Shift Arithmetic7/1
  Extract Bits15/1 -> Data Type Conversion21/1
  Bus Selector/7 -> Data Type Conversion20/1  "<RAW_Byte_7>"
  Data Type Conversion19/1 -> Add/14
  Shift Arithmetic6/1 -> Add/13
  Data Type Conversion20/1 -> Extract Bits14/1, Extract Bits13/1
  Data Type Conversion18/1 -> Shift Arithmetic6/1
  Extract Bits14/1 -> Data Type Conversion19/1
  Extract Bits13/1 -> Data Type Conversion18/1
  Bus Selector/6 -> Data Type Conversion17/1  "<RAW_Byte_6>"
  Data Type Conversion16/1 -> Add/12
  Shift Arithmetic5/1 -> Add/11
  Data Type Conversion17/1 -> Extract Bits11/1, Extract Bits12/1
  Data Type Conversion15/1 -> Shift Arithmetic5/1
  Extract Bits12/1 -> Data Type Conversion16/1
  Extract Bits11/1 -> Data Type Conversion15/1
  Bus Selector/5 -> Data Type Conversion14/1  "<RAW_Byte_5>"
  Data Type Conversion13/1 -> Add/10
  Shift Arithmetic4/1 -> Add/9
  Data Type Conversion14/1 -> Extract Bits9/1, Extract Bits10/1
  Data Type Conversion12/1 -> Shift Arithmetic4/1
  Extract Bits9/1 -> Data Type Conversion13/1
  Extract Bits10/1 -> Data Type Conversion12/1
  Bus Selector/4 -> Data Type Conversion9/1  "<RAW_Byte_4>"
  Data Type Conversion11/1 -> Add/8
  Shift Arithmetic3/1 -> Add/7
  Data Type Conversion9/1 -> Extract Bits8/1, Extract Bits7/1
  Data Type Conversion10/1 -> Shift Arithmetic3/1
  Extract Bits7/1 -> Data Type Conversion11/1
  Extract Bits8/1 -> Data Type Conversion10/1
  Bus Selector/3 -> Data Type Conversion6/1  "<RAW_Byte_3>"
  Data Type Conversion8/1 -> Add/6
  Shift Arithmetic2/1 -> Add/5
  Data Type Conversion6/1 -> Extract Bits5/1, Extract Bits6/1
  Data Type Conversion7/1 -> Shift Arithmetic2/1
  Extract Bits5/1 -> Data Type Conversion8/1
  Extract Bits6/1 -> Data Type Conversion7/1
  Bus Selector/2 -> Data Type Conversion3/1  "<RAW_Byte_2>"
  Data Type Conversion5/1 -> Add/4
  Shift Arithmetic1/1 -> Add/3
  Data Type Conversion2/1 -> Add/2
  Shift Arithmetic/1 -> Add/1
  Data Type Conversion3/1 -> Extract Bits4/1, Extract Bits3/1
  Data Type Conversion4/1 -> Shift Arithmetic1/1
  Extract Bits3/1 -> Data Type Conversion5/1
  Extract Bits4/1 -> Data Type Conversion4/1
  Data Type Conversion/1 -> Extract Bits1/1, Extract Bits2/1
  Data Type Conversion1/1 -> Shift Arithmetic/1
  Extract Bits1/1 -> Data Type Conversion2/1
  Extract Bits2/1 -> Data Type Conversion1/1
  Bus Selector/1 -> Data Type Conversion/1  "<RAW_Byte_1>"
